simulink model "dualConversionSuperheterodyneReceiver"  (R2021b)
settings: Solver=VariableStepAuto  StartTime=0.0  StopTime=10.0  RelTol=1e-3
undefined symbols (not defined in the file): fdesignblkfcn, gcbh
libraries: dsparch4 x6, dspsrcs4 x4
settings Model: Creator=Zireael  LastModifiedBy=Zireael

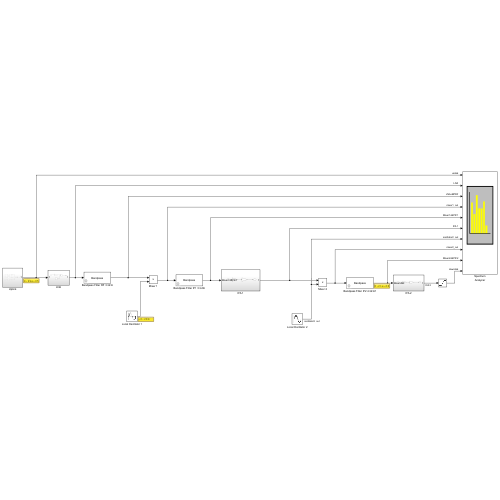
[thumbnail: Simulink's stored preview of the top-level diagram]
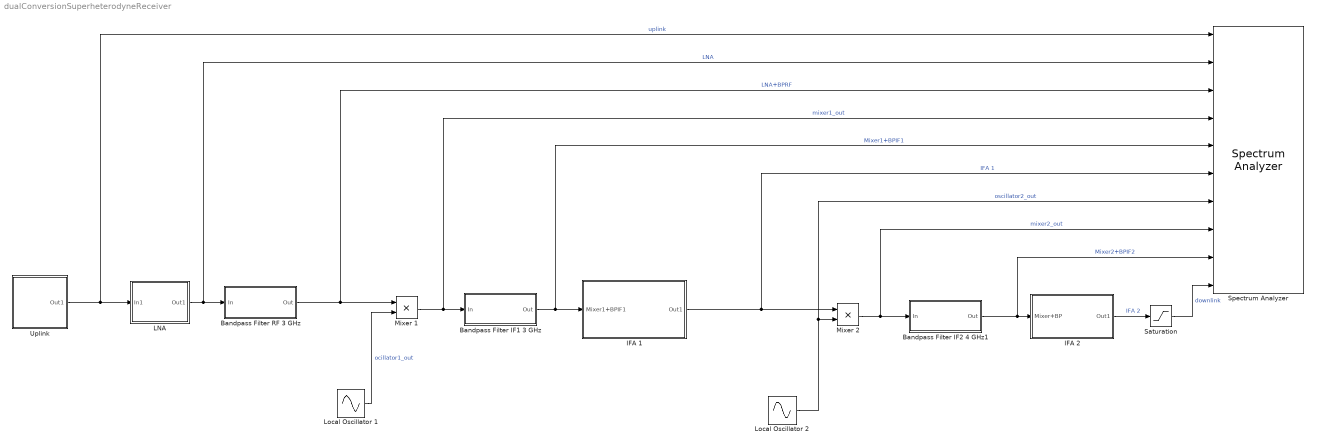
== system dualConversionSuperheterodyneReceiver ==
  Bandpass Filter IF1 3 GHz : Subsystem  DialogController=fdesignblkfcn  InitFcn=fdesignblkfcn(gcbh, {'InitFcn'});  mask(Bandpass Filter){}
      mask help: Design a bandpass filter
      settings: CopyFcn=fdesignblkfcn(gcbh, {'CopyFcn'});
      mask Help: helpview(mapfilelocation('dsp'), 'dspbandpassfilter');
      mask Display: disp('Bandpass');
  Bandpass Filter IF2 4 GHz1 : Subsystem  DialogController=fdesignblkfcn  InitFcn=fdesignblkfcn(gcbh, {'InitFcn'});  mask(Bandpass Filter){}
      mask help: Design a bandpass filter
      settings: CopyFcn=fdesignblkfcn(gcbh, {'CopyFcn'});
      mask Help: helpview(mapfilelocation('dsp'), 'dspbandpassfilter');
      mask Display: disp('Bandpass');
  Bandpass Filter RF 3 GHz : Subsystem  DialogController=fdesignblkfcn  InitFcn=fdesignblkfcn(gcbh, {'InitFcn'});  mask(Bandpass Filter){}
      mask help: Design a bandpass filter
      settings: CopyFcn=fdesignblkfcn(gcbh, {'CopyFcn'});
      mask Help: helpview(mapfilelocation('dsp'), 'dspbandpassfilter');
      mask Display: disp('Bandpass');
  IFA 1 : Subsystem
  IFA 2 : Subsystem
  LNA : Subsystem
  Local Oscillator 1 : Sin  Frequency=2*pi*2225e6  SampleTime=1/(50e9)
  Local Oscillator 2 : Sin  Frequency=2*pi*2225e6  SampleTime=1/(50e9)
  Mixer 1 : Product
  Mixer 2 : Product
  Saturation : Saturate  UpperLimit=0.9e4  LowerLimit=-0.9e4
  Spectrum Analyzer : SpectrumAnalyzer  NumInputPorts=10
  Uplink : Subsystem
  wires:
  Local Oscillator 1/1 -> Mixer 1/2  "ocillator1_out"
  Uplink/1(Out1) -> Spectrum Analyzer/1, LNA/1(In1)  "uplink"
  Bandpass Filter RF 3 GHz/1(Out) -> Spectrum Analyzer/3, Mixer 1/1  "LNA+BPRF"
  LNA/1(Out1) -> Spectrum Analyzer/2, Bandpass Filter RF 3 GHz/1(In)  "LNA"
  Mixer 1/1 -> Spectrum Analyzer/4, Bandpass Filter IF1 3 GHz/1(In)  "mixer1_out"
  Bandpass Filter IF1 3 GHz/1(Out) -> Spectrum Analyzer/5, IFA 1/1(Mixer1+BPIF1)  "Mixer1+BPIF1"
  Local Oscillator 2/1 -> Mixer 2/2, Spectrum Analyzer/7  "oscillator2_out"
  Mixer 2/1 -> Spectrum Analyzer/8, Bandpass Filter IF2 4 GHz1/1(In)  "mixer2_out"
  Bandpass Filter IF2 4 GHz1/1(Out) -> Spectrum Analyzer/9, IFA 2/1(Mixer+BP)  "Mixer2+BPIF2"
  IFA 1/1(Out1) -> Spectrum Analyzer/6, Mixer 2/1  "IFA 1"
  IFA 2/1(Out1) -> Saturation/1  "IFA 2"
  Saturation/1 -> Spectrum Analyzer/10  "downlink"

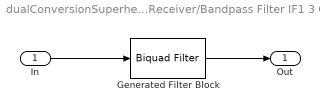
== system dualConversionSuperheterodyneReceiver/Bandpass Filter IF1 3 GHz ==
  In : Inport
  Generated Filter Block : dsparch4/Biquad Filter  Tag=BlockMethodSubSystem  FilterSource=Dialog parameters  CoeffSource=Specify via dialog  FilterObject=BQF  IIRFiltStruct=Direct form II  BiQuadCoeffs=[0.0474483370232056667 0 -0.0474483370232056667 1 -1.87473780518658106 0.994021428470330592;0.0156036763005154011 0 -0.0156036763005154011 1 -1.84168720614638048 0.993289491878398878;0.0104749993497772302 0 -0.0104749993497772302 1 -1.86043581304062422 0.99125783428283909;0.013298228938786268 0 -0.013298228938786268 1 -1.85308245656885529 0.991031691792957914;0.0681244127689580314 0 -0.0681244127689580314 1 -1.88471907472783684 0.998706960309933778;0.00942903498866506581 0 -0.00942903498866506581 1 -1.8391240977845178 0.9984801895777764;0.0237207251592587917 0 -0.0237207251592587917 1 -1.86787677139191821 0.992305622271925536;0.0115010399523870713 0 -0.0115010399523870713 1 -1.84657706227515606 0.991713591474610134;0.0636765532976010101 0 -0.0636765532976010101 1 -1.88048474343325767 0.996219447911953826;1.48894485140720056 0 -1.48894485140720056 1 -1.83906644505441941 0.995626810281686536]  ScaleValues=[0.00203991914968041418;1;1;1;1;1;1;1;1;1;1]  IC=0  ICnum=0  ICden=0  a0Flag=Warning  optimizeScaleValues=off  ScaleValueMode=Specify via input port (g)  InputProcessing=Columns as channels (frame based)  roundingMode=Floor  overflowMode=off  scaleValueFracLength=14  denProdOutputFracLength=30  denAccumFracLength=30  secondMemoryFracLength=15
  Out : Outport  VectorParamsAs1DForOutWhenUnconnected=off
  wires:
  In/1 -> Generated Filter Block/1
  Generated Filter Block/1 -> Out/1

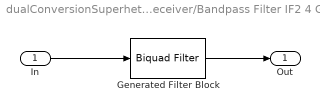
== system dualConversionSuperheterodyneReceiver/Bandpass Filter IF2 4 GHz1 ==
  In : Inport
  Generated Filter Block : dsparch4/Biquad Filter  Tag=BlockMethodSubSystem  FilterSource=Dialog parameters  CoeffSource=Specify via dialog  FilterObject=BQF  IIRFiltStruct=Direct form II  BiQuadCoeffs=[0.0474483370232056667 0 -0.0474483370232056667 1 -1.87473780518658106 0.994021428470330592;0.0156036763005154011 0 -0.0156036763005154011 1 -1.84168720614638048 0.993289491878398878;0.0104749993497772302 0 -0.0104749993497772302 1 -1.86043581304062422 0.99125783428283909;0.013298228938786268 0 -0.013298228938786268 1 -1.85308245656885529 0.991031691792957914;0.0681244127689580314 0 -0.0681244127689580314 1 -1.88471907472783684 0.998706960309933778;0.00942903498866506581 0 -0.00942903498866506581 1 -1.8391240977845178 0.9984801895777764;0.0237207251592587917 0 -0.0237207251592587917 1 -1.86787677139191821 0.992305622271925536;0.0115010399523870713 0 -0.0115010399523870713 1 -1.84657706227515606 0.991713591474610134;0.0636765532976010101 0 -0.0636765532976010101 1 -1.88048474343325767 0.996219447911953826;1.48894485140720056 0 -1.48894485140720056 1 -1.83906644505441941 0.995626810281686536]  ScaleValues=[0.00203991914968041418;1;1;1;1;1;1;1;1;1;1]  IC=0  ICnum=0  ICden=0  a0Flag=Warning  optimizeScaleValues=off  ScaleValueMode=Specify via input port (g)  InputProcessing=Columns as channels (frame based)  roundingMode=Floor  overflowMode=off  scaleValueFracLength=14  denProdOutputFracLength=30  denAccumFracLength=30  secondMemoryFracLength=15
  Out : Outport  VectorParamsAs1DForOutWhenUnconnected=off
  wires:
  In/1 -> Generated Filter Block/1
  Generated Filter Block/1 -> Out/1

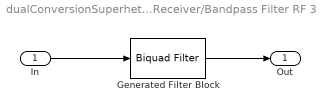
== system dualConversionSuperheterodyneReceiver/Bandpass Filter RF 3 GHz ==
  In : Inport
  Generated Filter Block : dsparch4/Biquad Filter  Tag=BlockMethodSubSystem  FilterSource=Dialog parameters  CoeffSource=Specify via dialog  FilterObject=BQF  IIRFiltStruct=Direct form II  BiQuadCoeffs=[0.0472672813008138265 0 -0.0472672813008138265 1 -1.85472128225473121 0.993992762161696186;0.0155639101151463406 0 -0.0155639101151463406 1 -1.81938169585511256 0.993318137905028875;0.0104595745355243568 0 -0.0104595745355243568 1 -1.83954209270283697 0.99124895401941493;0.0134791130640470758 0 -0.0134791130640470758 1 -1.83168724517741399 0.991040570110002128;0.0675394459376376932 0 -0.0675394459376376932 1 -1.86514793760057329 0.998698106447508449;0.0094309264239724102 0 -0.0094309264239724102 1 -1.81628872489633597 0.998489041508277109;0.0236072764525103555 0 -0.0236072764525103555 1 -1.84745707164067197 0.992282395639045189;0.0116677676085447241 0 -0.0116677676085447241 1 -1.82469717624845829 0.99173680479333115;0.0631166002369145385 0 -0.0631166002369145385 1 -1.86076147639443468 0.996196279984706834;1.37884728596692452 0 -1.37884728596692452 1 -1.81643207848185173 0.995649964965125922]  ScaleValues=[0.00220720158908927801;1;1;1;1;1;1;1;1;1;1]  IC=0  ICnum=0  ICden=0  a0Flag=Warning  optimizeScaleValues=off  ScaleValueMode=Specify via input port (g)  InputProcessing=Columns as channels (frame based)  roundingMode=Floor  overflowMode=off  scaleValueFracLength=14  denProdOutputFracLength=30  denAccumFracLength=30  secondMemoryFracLength=15
  Out : Outport  VectorParamsAs1DForOutWhenUnconnected=off
  wires:
  In/1 -> Generated Filter Block/1
  Generated Filter Block/1 -> Out/1

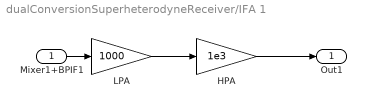
== system dualConversionSuperheterodyneReceiver/IFA 1 ==
  Mixer1+BPIF1 : Inport
  HPA : Gain  Gain=1e3
  LPA : Gain  Gain=1000
  Out1 : Outport
  wires:
  Mixer1+BPIF1/1 -> LPA/1
  LPA/1 -> HPA/1
  HPA/1 -> Out1/1

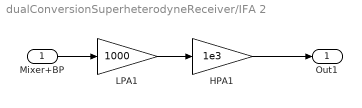
== system dualConversionSuperheterodyneReceiver/IFA 2 ==
  Mixer+BP : Inport
  HPA1 : Gain  Gain=1e3
  LPA1 : Gain  Gain=1000
  Out1 : Outport
  wires:
  LPA1/1 -> HPA1/1
  HPA1/1 -> Out1/1
  Mixer+BP/1 -> LPA1/1

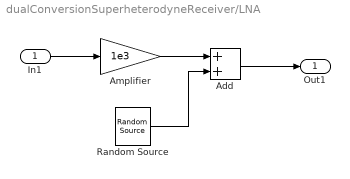
== system dualConversionSuperheterodyneReceiver/LNA ==
  In1 : Inport
  Add : Sum
  Amplifier : Gain  Gain=1e3
  Random Source : dspsrcs4/Random Source  SrcType=Gaussian  NormMethod=Ziggurat  CltLength=12  MinVal=0  MaxVal=1  MeanVal=0  VarVal=1e-3  RepMode=Not repeatable  rawSeed=1  IsInherit=off  SampMode=Discrete  SampTime=1/(50e9)  SampFrame=1  DataType=Double  OutComplex=Real  OutputFrames=off
  Out1 : Outport
  wires:
  Random Source/1 -> Add/2
  Amplifier/1 -> Add/1
  Add/1 -> Out1/1
  In1/1 -> Amplifier/1

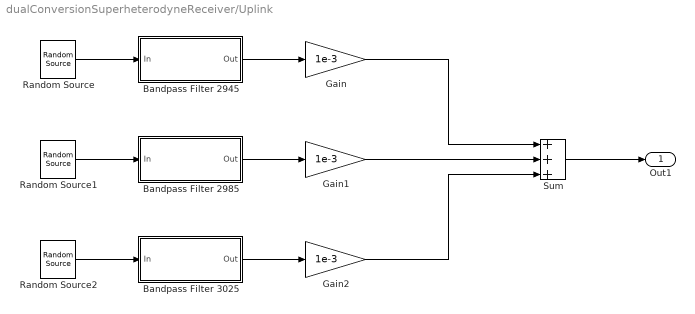
== system dualConversionSuperheterodyneReceiver/Uplink ==
  Bandpass Filter 2945 : Subsystem  DialogController=fdesignblkfcn  InitFcn=fdesignblkfcn(gcbh, {'InitFcn'});  mask(Bandpass Filter){}
      mask help: Design a bandpass filter
      settings: CopyFcn=fdesignblkfcn(gcbh, {'CopyFcn'});
      mask Help: helpview(mapfilelocation('dsp'), 'dspbandpassfilter');
      mask Display: disp('Bandpass');
  Bandpass Filter 2985 : Subsystem  DialogController=fdesignblkfcn  InitFcn=fdesignblkfcn(gcbh, {'InitFcn'});  mask(Bandpass Filter){}
      mask help: Design a bandpass filter
      settings: CopyFcn=fdesignblkfcn(gcbh, {'CopyFcn'});
      mask Help: helpview(mapfilelocation('dsp'), 'dspbandpassfilter');
      mask Display: disp('Bandpass');
  Bandpass Filter 3025 : Subsystem  DialogController=fdesignblkfcn  InitFcn=fdesignblkfcn(gcbh, {'InitFcn'});  mask(Bandpass Filter){}
      mask help: Design a bandpass filter
      settings: CopyFcn=fdesignblkfcn(gcbh, {'CopyFcn'});
      mask Help: helpview(mapfilelocation('dsp'), 'dspbandpassfilter');
      mask Display: disp('Bandpass');
  Gain : Gain  Gain=1e-3
  Gain1 : Gain  Gain=1e-3
  Gain2 : Gain  Gain=1e-3
  Random Source : dspsrcs4/Random Source  SrcType=Gaussian  NormMethod=Ziggurat  CltLength=12  MinVal=0  MaxVal=1  MeanVal=0  VarVal=1  RepMode=Not repeatable  rawSeed=1  IsInherit=off  SampMode=Discrete  SampTime=1/(50e9)  SampFrame=1  DataType=Double  OutComplex=Real  OutputFrames=off
  Random Source1 : dspsrcs4/Random Source  SrcType=Gaussian  NormMethod=Ziggurat  CltLength=12  MinVal=0  MaxVal=1  MeanVal=0  VarVal=1  RepMode=Not repeatable  rawSeed=1  IsInherit=off  SampMode=Discrete  SampTime=1/(50e9)  SampFrame=1  DataType=Double  OutComplex=Real  OutputFrames=off
  Random Source2 : dspsrcs4/Random Source  SrcType=Gaussian  NormMethod=Ziggurat  CltLength=12  MinVal=0  MaxVal=1  MeanVal=0  VarVal=1  RepMode=Not repeatable  rawSeed=1  IsInherit=off  SampMode=Discrete  SampTime=1/(50e9)  SampFrame=1  DataType=Double  OutComplex=Real  OutputFrames=off
  Sum : Sum  Inputs=+++
  Out1 : Outport
  wires:
  Random Source/1 -> Bandpass Filter 2945/1(In)
  Bandpass Filter 2945/1(Out) -> Gain/1
  Bandpass Filter 2985/1(Out) -> Gain1/1
  Random Source1/1 -> Bandpass Filter 2985/1(In)
  Random Source2/1 -> Bandpass Filter 3025/1(In)
  Bandpass Filter 3025/1(Out) -> Gain2/1
  Sum/1 -> Out1/1
  Gain/1 -> Sum/1
  Gain1/1 -> Sum/2
  Gain2/1 -> Sum/3

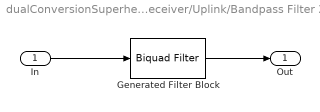
== system dualConversionSuperheterodyneReceiver/Uplink/Bandpass Filter 2945 ==
  In : Inport
  Generated Filter Block : dsparch4/Biquad Filter  Tag=BlockMethodSubSystem  FilterSource=Dialog parameters  CoeffSource=Specify via dialog  FilterObject=BQF  IIRFiltStruct=Direct form II  BiQuadCoeffs=[0.00391109570396021029 0 -0.00391109570396021029 1 -1.86581793613173952 0.999785458346093336;0.00146314559405021191 0 -0.00146314559405021191 1 -1.86296930405197303 0.999783271073049873;0.00113593867170552515 0 -0.00113593867170552515 1 -1.86455035007572123 0.999578709207089688;0.000964094221033681134 0 -0.000964094221033681134 1 -1.86386607203634247 0.999577682125649125;0.00173389847257807736 0 -0.00173389847257807736 1 -1.86524035067752747 0.999652318157665976;0.000850606119426623058 0 -0.000850606119426623058 1 -1.863306223531219 0.999649916422154838;0.00420661380233906118 0 -0.00420661380233906118 1 -1.86618519059587973 0.999955178758414776;0.000273525583557842668 0 -0.000273525583557842668 1 -1.86291545489429233 0.999954653561259899;0.00362913638073846835 0 -0.00362913638073846835 1 -1.86554999745247807 0.999712689702571877;0.0013326548585498321 0 -0.0013326548585498321 1 -1.86310506283457711 0.999710178066045674;0.000654726137269481595 0 -0.000654726137269481595 1 -1.86419984341850009 0.999568774242084457;0.00136330267483060529 0 -0.00136330267483060529 1 -1.86490227598014058 0.999606986964023836;0.00116234133070601433 0 -0.00116234133070601433 1 -1.86356372884863308 0.99960511035788624;0.00402094440234465871 0 -0.00402094440234465871 1 -1.86603271995711983 0.999867467004967647;1.38242446731734514 0 -1.38242446731734514 1 -1.86290511316609253 0.999865982352868388]  ScaleValues=[8.37752633663082981e-05;1;1;1;1;1;1;1;1;1;1;1;1;1;1;1]  IC=0  ICnum=0  ICden=0  a0Flag=Warning  optimizeScaleValues=off  ScaleValueMode=Specify via input port (g)  InputProcessing=Columns as channels (frame based)  roundingMode=Floor  overflowMode=off  scaleValueFracLength=14  denProdOutputFracLength=30  denAccumFracLength=30  secondMemoryFracLength=15
  Out : Outport  VectorParamsAs1DForOutWhenUnconnected=off
  wires:
  In/1 -> Generated Filter Block/1
  Generated Filter Block/1 -> Out/1

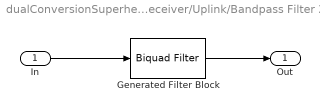
== system dualConversionSuperheterodyneReceiver/Uplink/Bandpass Filter 2985 ==
  In : Inport
  Generated Filter Block : dsparch4/Biquad Filter  Tag=BlockMethodSubSystem  FilterSource=Dialog parameters  CoeffSource=Specify via dialog  FilterObject=BQF  IIRFiltStruct=Direct form II  BiQuadCoeffs=[0.00395233271133889341 0 -0.00395233271133889341 1 -1.86217710033880968 0.999785442251455603;0.00150403688841968227 0 -0.00150403688841968227 1 -1.85929165601175095 0.999783287167650192;0.00116075382481968655 0 -0.00116075382481968655 1 -1.86089588664867533 0.999578701649000867;0.000923745960181922049 0 -0.000923745960181922049 1 -1.86020277943418599 0.999577689683735615;0.00177498468711014662 0 -0.00177498468711014662 1 -1.86159382963987374 0.999652300485325163;0.000817391174800780507 0 -0.000817391174800780507 1 -1.85963473309039062 0.999649934094456682;0.00228454912414921248 0 -0.00228454912414921248 1 -1.86254679535119072 0.999955174893824905;0.000575149692407939095 0 -0.000575149692407939095 1 -1.85923475118582138 0.999954657425852322;0.00345108790955189065 0 -0.00345108790955189065 1 -1.8619066742975332 0.99971267122139984;0.00134512247724787081 0 -0.00134512247724787081 1 -1.8594301615856117 0.999710196547167196;0.000623029390963172739 0 -0.000623029390963172739 1 -1.8605409818270453 0.999568774242084235;0.00143015479887003815 0 -0.00143015479887003815 1 -1.86125198667097447 0.999606973158225665;0.00111099834102953857 0 -0.00111099834102953857 1 -1.85989616481269282 0.99960512416366154;0.00414775614930111645 0 -0.00414775614930111645 1 -1.86239355147126351 0.999867456080969497;1.37085125887247639 0 -1.37085125887247639 1 -1.85922550225031502 0.999865993276849219]  ScaleValues=[7.82704829772785129e-05;1;1;1;1;1;1;1;1;1;1;1;1;1;1;1]  IC=0  ICnum=0  ICden=0  a0Flag=Warning  optimizeScaleValues=off  ScaleValueMode=Specify via input port (g)  InputProcessing=Columns as channels (frame based)  roundingMode=Floor  overflowMode=off  scaleValueFracLength=14  denProdOutputFracLength=30  denAccumFracLength=30  secondMemoryFracLength=15
  Out : Outport  VectorParamsAs1DForOutWhenUnconnected=off
  wires:
  In/1 -> Generated Filter Block/1
  Generated Filter Block/1 -> Out/1

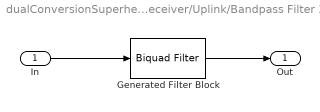
== system dualConversionSuperheterodyneReceiver/Uplink/Bandpass Filter 3025 ==
  In : Inport
  Generated Filter Block : dsparch4/Biquad Filter  Tag=BlockMethodSubSystem  FilterSource=Dialog parameters  CoeffSource=Specify via dialog  FilterObject=BQF  IIRFiltStruct=Direct form II  BiQuadCoeffs=[0.0041219989158373339 0 -0.0041219989158373339 1 -1.85866777616438794 0.999876944623845798;0.000829112268078909995 0 -0.000829112268078909995 1 -1.85555728499306349 0.999875647434137482;0.00275347631762093512 0 -0.00275347631762093512 1 -1.85785693352338521 0.999725217885755302;0.000721796128793744792 0 -0.000721796128793744792 1 -1.85609711117206788 0.999723583556367479;0.00117486705796178447 0 -0.00117486705796178447 1 -1.8573363476439031 0.999686122496876273;0.000752226893558737898 0 -0.000752226893558737898 1 -1.85655000489694388 0.999685289791654719;0.00297372344799259761 0 -0.00297372344799259761 1 -1.85831543341217564 0.999790977926174218;0.000657060530529696022 0 -0.000657060530529696022 1 -1.85575474917680183 0.999789166152854403;0.00325716009378984681 0 -0.00325716009378984681 1 -1.85888027605336958 0.999974780053434875;0.000145054753481166007 0 -0.000145054753481166007 1 -1.85552474529498701 0.999974493047233959;0.00395835391432667553 0 -0.00395835391432667553 1 -1.85850726373241382 0.999831921169928028;0.00114435556037660764 0 -0.00114435556037660764 1 -1.85563628284949655 0.9998302866849611;0.00288261554021760572 0 -0.00288261554021760572 1 -1.85760134486320672 0.999702025723047116;0.000924716345314715205 0 -0.000924716345314715205 1 -1.85631235667384198 0.999700728737886513;0.000642949504821922519 0 -0.000642949504821922519 1 -1.85706841536069156 0.999677916470901096;0.00102335090816065748 0 -0.00102335090816065748 1 -1.85680412660172056 0.99967762955938555;0.00212720825557144097 0 -0.00212720825557144097 1 -1.85809689952402324 0.999755116006149636;0.00119294314835138989 0 -0.00119294314835138989 1 -1.8559096669187547 0.999753304290917244;0.00380961166046796121 0 -0.00380961166046796121 1 -1.85879311650978374 0.999924952497828534;1.34682069371837287 0 -1.34682069371837287 1 -1.85551978068988266 0.999924119612309426]  ScaleValues=[8.02185569867322728e-05;1;1;1;1;1;1;1;1;1;1;1;1;1;1;1;1;1;1;1;1]  IC=0  ICnum=0  ICden=0  a0Flag=Warning  optimizeScaleValues=off  ScaleValueMode=Specify via input port (g)  InputProcessing=Columns as channels (frame based)  roundingMode=Floor  overflowMode=off  scaleValueFracLength=14  denProdOutputFracLength=30  denAccumFracLength=30  secondMemoryFracLength=15
  Out : Outport  VectorParamsAs1DForOutWhenUnconnected=off
  wires:
  Generated Filter Block/1 -> Out/1
  In/1 -> Generated Filter Block/1
